simulink model "my_pv_sys_fpga"  (Simulink 8.4)
settings: Solver=ode3  StartTime=0.0  StopTime=10.0  RelTol=1e-3
undefined symbols (not defined in the file or in its folder): Ts
libraries: powerlib x30
settings Model: Creator=jiang  LastModifiedBy=jiang
settings DataIOCC: SignalLoggingSaveFormat=Dataset
settings OptimizationCC: ExpressionDepthLimit=128
settings DebuggingCC: UnderspecifiedInitializationDetection=Simplified  MergeDetectMultiDrivingBlocksExec=error  FcnCallInpInsideContextMsg=EnableAllAsError  StateNameClashWarn=none
settings GRTTargetCC: CombineOutputUpdateFcns=on  GRTInterface=off

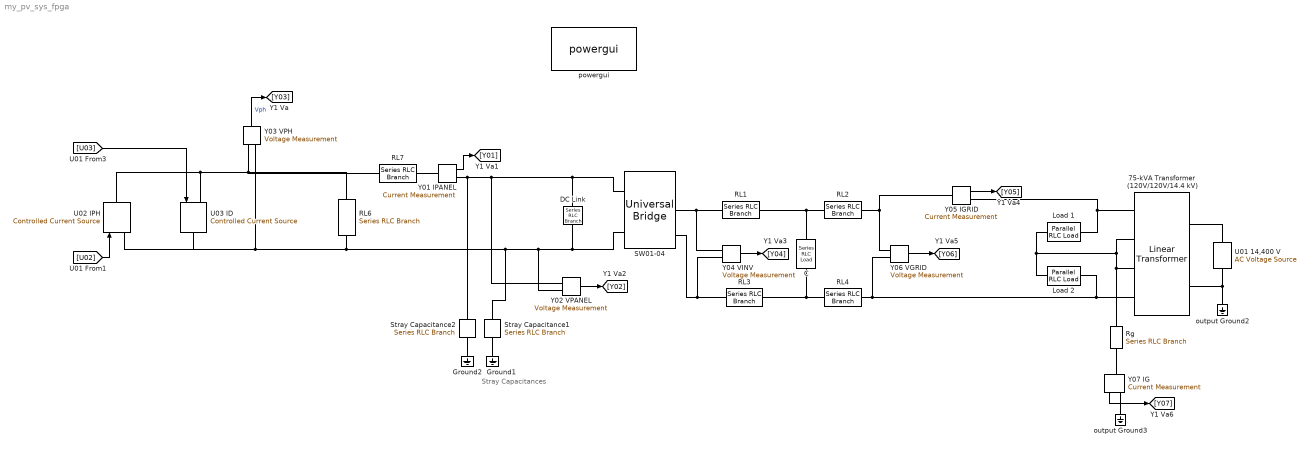
== system my_pv_sys_fpga ==
  note: Stray
      | Capacitances
  75-kVA Transformer (120V/120V/14.4 kV) : powerlib/Elements/Linear Transformer  UNITS=pu  NominalPower=[75e3,60]  winding1=[14.4e3 0.01,0.03]  winding2=[120,0.02,0]  ThreeWindings=on  winding3=[120,0.02,0]  RmLm=[50,50]  Measurements=None  DataType=off
  C : powerlib/Elements/Series RLC Load  LConnTagsString=a  RConnTagsString=__new0  NominalVoltage=240  NominalFrequency=50  ActivePower=10.5  InductivePower=0  CapacitivePower=525  Setx0=off  InitialVoltage=0  SetiL0=off  InitialCurrent=0  Measurements=None
  DC Link : powerlib/Elements/Series RLC Branch  LConnTagsString=__new0  RConnTagsString=__new0  BranchType=C  Resistance=1.0  Inductance=1.0  SetiL0=off  InitialCurrent=0  Capacitance=3000e-6  Setx0=on  InitialVoltage=400  Measurements=None
  Ground1 : powerlib/Elements/Ground  LConnTagsString=a
  Ground2 : powerlib/Elements/Ground  LConnTagsString=a
  Load 1 : powerlib/Elements/Parallel RLC Load  LConnTagsString=a  RConnTagsString=__new0  NominalVoltage=120  NominalFrequency=50  ActivePower=5e3  InductivePower=2e3  CapacitivePower=0  Setx0=off  InitialVoltage=0  SetiL0=off  InitialCurrent=0  Measurements=None
      settings: AttributesFormatString=\n
  Load 2 : powerlib/Elements/Parallel RLC Load  LConnTagsString=a  RConnTagsString=__new0  NominalVoltage=120  NominalFrequency=50  ActivePower=5e3  InductivePower=2e3  CapacitivePower=0  Setx0=off  InitialVoltage=0  SetiL0=off  InitialCurrent=0  Measurements=None
      settings: AttributesFormatString=\n
  RL{1..4} (4 alike) : powerlib/Elements/Series RLC Branch  LConnTagsString=__new0  RConnTagsString=__new0  BranchType=RL  Resistance=8.23e-3  Inductance=2.183e-3  SetiL0=off  InitialCurrent=0  Capacitance=1e-6  Setx0=off  InitialVoltage=0  Measurements=None
  RL6 : powerlib/Elements/Series RLC Branch  LConnTagsString=__new0  RConnTagsString=__new0  BranchType=R  Resistance=301.8*14  Inductance=2.183e-3  SetiL0=off  InitialCurrent=0  Capacitance=1e-6  Setx0=off  InitialVoltage=0  Measurements=None
  RL7 : powerlib/Elements/Series RLC Branch  LConnTagsString=__new0  RConnTagsString=__new0  BranchType=R  Resistance=0.247*14  Inductance=2.183e-3  SetiL0=off  InitialCurrent=0  Capacitance=1e-6  Setx0=off  InitialVoltage=0  Measurements=None
  Rg : powerlib/Elements/Series RLC Branch  LConnTagsString=__new0  RConnTagsString=__new0  BranchType=R  Resistance=0.2  Inductance=1  SetiL0=off  InitialCurrent=0  Capacitance=50e-9  Setx0=off  InitialVoltage=0  Measurements=None
  SW01-04 : powerlib/Power Electronics/Universal Bridge  Arms=2  SnubberResistance=1e6  SnubberCapacitance=inf  Device=IGBT / Diodes  Ron=1e-3  Lon=0  ForwardVoltages=[ 0 0 ]  ForwardVoltage=0  GTOparameters=[ 10e-6 , 20e-6 ]  IGBTparameters=[ 50e-6 , 50e-6 ]*0  Measurements=None  Measurements_2=None  converterType=Rectifier
  Stray Capacitance1 : powerlib/Elements/Series RLC Branch  LConnTagsString=__new0  RConnTagsString=__new0  BranchType=C  Resistance=1e-3  Inductance=1  SetiL0=off  InitialCurrent=0  Capacitance=4e-9  Setx0=off  InitialVoltage=0  Measurements=None
  Stray Capacitance2 : powerlib/Elements/Series RLC Branch  LConnTagsString=__new0  RConnTagsString=__new0  BranchType=C  Resistance=1e-3  Inductance=1  SetiL0=off  InitialCurrent=0  Capacitance=4e-9  Setx0=off  InitialVoltage=0  Measurements=None
  U01 14,400 V : powerlib/Electrical Sources/AC Voltage Source  Description=source block  Amplitude=14400*sqrt(2)  Phase=0  Frequency=50  SampleTime=0  Measurements=None
      settings: AttributesFormatString=\n
  "U02 IPH " : powerlib/Electrical Sources/Controlled Current Source  Initialize=on  Source_Type=DC  Amplitude=8.05  Phase=0  Frequency=0  Measurements=None
  "U03 ID " : powerlib/Electrical Sources/Controlled Current Source  Initialize=on  Source_Type=DC  Amplitude=8.05  Phase=0  Frequency=0  Measurements=None
  Y01 IPANEL : powerlib/Measurements/Current Measurement  PhasorSimulation=off  OutputType=Complex  PSBequivalent=0
  Y02 VPANEL : powerlib/Measurements/Voltage Measurement  PhasorSimulation=off  OutputType=Complex  PSBequivalent=0
  Y03 VPH : powerlib/Measurements/Voltage Measurement  PhasorSimulation=off  OutputType=Complex  PSBequivalent=0
  Y04 VINV : powerlib/Measurements/Voltage Measurement  PhasorSimulation=off  OutputType=Complex  PSBequivalent=0
  Y05 IGRID : powerlib/Measurements/Current Measurement  PhasorSimulation=off  OutputType=Complex  PSBequivalent=0
  Y06 VGRID : powerlib/Measurements/Voltage Measurement  PhasorSimulation=off  OutputType=Complex  PSBequivalent=0
  Y07 IG : powerlib/Measurements/Current Measurement  PhasorSimulation=off  OutputType=Complex  PSBequivalent=0
  output Ground2 : powerlib/Elements/Ground  LConnTagsString=a
  output Ground3 : powerlib/Elements/Ground  LConnTagsString=a
  powergui : powerlib/powergui  Priority=1  SimulationMode=Discrete  SolverType=Tustin/Backward Euler (TBE)  SampleTime=Ts  frequency=60  SPID=off  DisableSnubberDevices=off  DisableRonSwitches=off  DisableVfSwitches=off  SwTol=0  DisplayEquations=off  Interpol=off  methode=off  Ts=0  frequencyindice=0  Pbase=100e6  ErrMax=1e-4  Iterations=50  UnitsV=kV  UnitsW=MW  FunctionMessages=off  echomessages=off  HookPort=off  EnableUseOfTLC=off  x0status=blocks  RestoreLinks=warning  ResistiveCurrentMeasurement=off  Frange=[0:2:500]  Ylog=off  Xlog=on  ShowGrid=off  save=off  variable=ZData  structure=ScopeData  ZoomFFT=off  StartTime=7.29  cycles=3  DisplayStyle=1  fundamental=50  FreqAxis=off  MaxFrequency=1000  frequencyindicesteady=1  RmsSteady=1  display=off
  wires:
  [U02] -> "U02 IPH "/1
  [U03] -> "U03 ID "/1
  Y03 VPH/1 -> [Y03]  "Vph"
  Y01 IPANEL/1 -> [Y01]
  Y02 VPANEL/1 -> [Y02]
  Y04 VINV/1 -> [Y04]
  Y05 IGRID/1 -> [Y05]
  Y06 VGRID/1 -> [Y06]
  Y07 IG/1 -> [Y07]
  connections:
  SW01-04/LConn1 -- Y04 VINV/LConn1 -- RL1/LConn1
  RL3/LConn1 -- Y04 VINV/LConn2 -- SW01-04/LConn2
  RL2/LConn1 -- C/RConn1 -- RL1/RConn1
  RL3/RConn1 -- RL4/LConn1 -- C/LConn1
  U01 14,400 V/LConn1 -- 75-kVA Transformer (120V/120V/14.4 kV)/LConn2 -- output Ground2/LConn1
  Y06 VGRID/LConn2 -- RL4/RConn1 -- Load 2/RConn1 -- 75-kVA Transformer (120V/120V/14.4 kV)/RConn4
  Load 1/RConn1 -- Y05 IGRID/RConn1 -- 75-kVA Transformer (120V/120V/14.4 kV)/RConn1
  75-kVA Transformer (120V/120V/14.4 kV)/RConn3 -- Rg/LConn1 -- 75-kVA Transformer (120V/120V/14.4 kV)/RConn2 -- Load 2/LConn1 -- Load 1/LConn1
  Ground2/LConn1 -- Stray Capacitance2/RConn1
  Y07 IG/LConn1 -- Rg/RConn1
  Ground1/LConn1 -- Stray Capacitance1/RConn1
  U01 14,400 V/RConn1 -- 75-kVA Transformer (120V/120V/14.4 kV)/LConn1
  Y07 IG/RConn1 -- output Ground3/LConn1
  DC Link/RConn1 -- Stray Capacitance1/LConn1 -- Y03 VPH/LConn2 -- "U03 ID "/RConn1 -- "U02 IPH "/LConn1 -- RL6/LConn1 -- Y02 VPANEL/LConn2 -- SW01-04/RConn2
  DC Link/LConn1 -- SW01-04/RConn1 -- Y02 VPANEL/LConn1 -- Stray Capacitance2/LConn1 -- Y01 IPANEL/RConn1
  RL7/RConn1 -- Y01 IPANEL/LConn1
  RL6/RConn1 -- RL7/LConn1 -- Y03 VPH/LConn1 -- "U03 ID "/LConn1 -- "U02 IPH "/RConn1
  Y05 IGRID/LConn1 -- Y06 VGRID/LConn1 -- RL2/RConn1
